simulink subsystem "INS_subs"  (R2021a)
settings: Solver=VariableStepAuto  StartTime=0.0  StopTime=10.0  RelTol=1e-3
libraries: simulink_extras x5
settings Model: Creator=kubab  LastModifiedBy=kubab

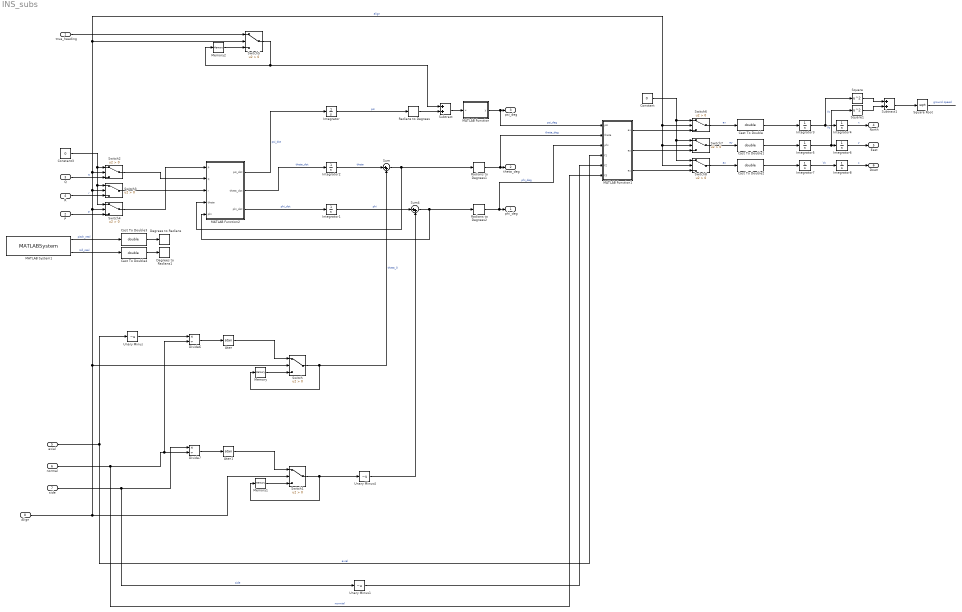
== system INS_subs ==
  true_heading : Inport
  P : Inport  Port=2
  Q : Inport  Port=3
  R : Inport  Port=4
  axial : Inport  Port=5
  normal : Inport  Port=6
  side : Inport  Port=7
  Align : Inport  Port=8
  Atan : Trigonometry  Operator=atan
  Atan1 : Trigonometry  Operator=atan
  Cast To Double{,1..4} (5 alike) : DataTypeConversion  OutDataTypeStr=double
  Constant : Constant  Value=0
  Constant3 : Constant  Value=0
  Degrees to Radians : simulink_extras/Transformations/Degrees to Radians
  Degrees to Radians1 : simulink_extras/Transformations/Degrees to Radians
  Divide6 : Product  Inputs=*/
  Divide7 : Product  Inputs=*/
  Integrator : Integrator  WrapState=on
  Integrator1 : Integrator  WrapState=on
  Integrator2 : Integrator  ContinuousStateAttributes='thwow'
  Integrator{3..8} (6 alike) : Integrator
  MATLAB Function : MATLAB Function  TreatAsAtomicUnit=on
  MATLAB Function1 : MATLAB Function  TreatAsAtomicUnit=on
  MATLAB Function2 : MATLAB Function  TreatAsAtomicUnit=on
  MATLAB System1 : MATLABSystem  System=Angles_real  SimulateUsing=Code generation
      mask Type: Angles_real
      mask Display:
      | disp('Angles_real');
      | port_label('output',1,'pitch');
      | port_label('output',2,'true_heading');
      | port_label('output',3,'roll');
  Memory : Memory
  Memory1 : Memory
  Memory2 : Memory
  Radians to Degrees : simulink_extras/Transformations/Radians to Degrees
  Radians to Degrees1 : simulink_extras/Transformations/Radians to Degrees
  Radians to Degrees2 : simulink_extras/Transformations/Radians to Degrees
  Square : Math  Operator=square  SaturateOnIntegerOverflow=on
  Square Root : Sqrt  SaturateOnIntegerOverflow=on
  Square1 : Math  Operator=square  SaturateOnIntegerOverflow=on
  Subtract : Sum
  Subtract1 : Sum
  Sum : Sum  Inputs=|++
  Sum4 : Sum  Inputs=|++
  Switch{,1..8} (9 alike) : Switch  Criteria=u2 > Threshold
  Unary Minus : UnaryMinus
  Unary Minus1 : UnaryMinus
  Unary Minus4 : UnaryMinus
  phi_deg : Outport
  theta_deg : Outport  Port=2
  psi_deg : Outport  Port=3
  North : Outport  Port=4
  East : Outport  Port=5
  Down : Outport  Port=6
  wires:
  P/1 -> Switch4/3  "p"
  Integrator2/1 -> Sum/1  "theta"
  normal/1 -> Divide7/2, Divide6/2, MATLAB Function1/6(f3)  "normial"
  Sum/1 -> Radians to Degrees1/1, MATLAB Function2/4(theta)
  MATLAB Function2/3(phi_dot) -> Integrator1/1  "phi_dot"
  Sum4/1 -> MATLAB Function2/5(phi), Radians to Degrees2/1
  Divide7/1 -> Atan1/1
  Align/1 -> Switch/2, Switch4/2, Switch3/2, Switch2/2, Switch6/2, Switch7/2, Switch8/2, Switch5/2, Switch1/2  "align"
  Switch1/1 -> Memory1/1, Unary Minus4/1
  Atan1/1 -> Switch1/1
  Memory1/1 -> Switch1/3
  Q/1 -> Switch2/3  "q"
  Constant3/1 -> Switch2/1, Switch3/1, Switch4/1
  Atan/1 -> Switch/1
  Divide6/1 -> Atan/1
  Memory/1 -> Switch/3
  Radians to Degrees1/1 -> theta_deg/1, MATLAB Function1/2(theta)  "theta_deg"
  Switch/1 -> Sum/2, Memory/1  "theta_0"
  MATLAB Function2/1(psi_dot) -> Integrator/1  "psi_dot"
  MATLAB Function2/2(theta_dot) -> Integrator2/1  "theta_dot"
  R/1 -> Switch3/3  "r"
  true_heading/1 -> Switch5/1
  Switch5/1 -> Memory2/1, Subtract/1
  Memory2/1 -> Switch5/3
  Radians to Degrees/1 -> Subtract/2
  MATLAB Function/1(y) -> psi_deg/1, MATLAB Function1/1(psi)  "psi_deg"
  Radians to Degrees2/1 -> phi_deg/1, MATLAB Function1/3(phi)  "phi_deg"
  Integrator1/1 -> Sum4/1  "phi"
  Integrator/1 -> Radians to Degrees/1  "psi"
  Subtract/1 -> MATLAB Function/1(u)
  MATLAB Function1/1(ax) -> Switch6/3
  MATLAB Function1/2(ay) -> Switch7/3
  MATLAB Function1/3(az) -> Switch8/3
  axial/1 -> Unary Minus/1, MATLAB Function1/4(f1)  "axial"
  Integrator3/1 -> Square/1, Integrator4/1  "Vx"
  Integrator7/1 -> Integrator8/1  "Vz"
  Integrator8/1 -> Down/1  "z"
  Integrator6/1 -> East/1  "y"
  Integrator4/1 -> North/1  "x"
  Unary Minus/1 -> Divide6/1
  Cast To Double1/1 -> Integrator5/1
  Cast To Double/1 -> Integrator3/1
  Unary Minus4/1 -> Sum4/2
  side/1 -> Divide7/1, Unary Minus1/1  "side"
  Cast To Double2/1 -> Integrator7/1
  Integrator5/1 -> Integrator6/1, Square1/1  "Vy"
  Square/1 -> Subtract1/1
  Square1/1 -> Subtract1/2
  Subtract1/1 -> Square Root/1
  Square Root/1 -> ?  "ground speed"
  Switch4/1 -> MATLAB Function2/1(p)
  Switch2/1 -> MATLAB Function2/2(q)
  Switch3/1 -> MATLAB Function2/3(r)
  Unary Minus1/1 -> MATLAB Function1/5(f2)
  Switch6/1 -> Cast To Double/1  "ax"
  Switch8/1 -> Cast To Double2/1  "az"
  Switch7/1 -> Cast To Double1/1  "ay"
  Constant/1 -> Switch7/1, Switch8/1, Switch6/1
  MATLAB System1/3 -> Cast To Double4/1  "roll_real"
  MATLAB System1/1 -> Cast To Double3/1  "pitch_real"
  Cast To Double3/1 -> Degrees to Radians/1
  Cast To Double4/1 -> Degrees to Radians1/1

== matlab function INS_subs/MATLAB Function1 ==
  data: ax output; psi input; theta input; phi input; ay output; az output; f1 input; f2 input; f3 input
function [ax, ay, az] = fcn(psi, theta, phi, f1, f2, f3)

g = 9.8065;

psi_rad = deg2rad(psi);
theta_rad = deg2rad(theta);
phi_rad = deg2rad(phi);

psi_matrix = [cos(psi_rad), -sin(psi_rad), 0;
              sin(psi_rad), cos(psi_rad), 0;
              0, 0, 1];
          
theta_matrix = [cos(theta_rad), 0, sin(theta_rad);
                0, 1, 0;
                -sin(theta_rad), 0, cos(theta_rad)];
           
phi_matrix = [1, 0, 0;
              0, cos(phi_rad), -sin(phi_rad);
              0, sin(phi_rad), cos(phi_rad)];

acc_input_matrix = [f1;f2;f3];

G = [0;0;-1];

acc_output_matrix = psi_matrix * theta_matrix * phi_matrix * acc_input_matrix + G;

ax = -acc_output_matrix(1,1) * g;
ay = -acc_output_matrix(2,1) * g;
az = -acc_output_matrix(3,1) * g;

== matlab function INS_subs/MATLAB Function ==
  data: u input; y output
function y = fcn(u)

    if u > 360
        y = u - 360;
    elseif u < 0
        y = u + 360;
    else
        y = u;
    end
end

== matlab function INS_subs/MATLAB Function2 ==
  data: p input; psi_dot output; q input; r input; theta input; phi input; theta_dot output; phi_dot output
function [psi_dot, theta_dot, phi_dot] = transform(p, q, r, theta, phi)

transform = [1, sin(phi)*tan(theta), cos(phi)*tan(theta);
             0, cos(phi), -sin(phi);
             0, sin(phi)/cos(theta), cos(phi)/cos(theta)];

angVel = transform*[p;q;r];

phi_dot = angVel(1);
theta_dot = angVel(2);
psi_dot = angVel(3);
